simulink model "H250Model"  (R2022a)
settings: Solver=ode4  StartTime=0.0  StopTime=inf  FixedStep=Ts  RelTol=1e-3
values from neighbouring files (symbols this model uses):
  ModelFail_env_P_wind = [0 0 0]    [F450DegradedParamInit.m]    (also in H250DegradedParamInit.m; H250ModelParam4S.m; H333DegradedParamInit4S.m)
  ModelFail_motor_isEnable = 0    [F450DegradedParamInit.m]    (also in H250DegradedParamInit.m; H250ModelParam4S.m; H333DegradedParamInit4S.m)
  ModelFail_motor_kCt = [1 1 1 1 1 1 1 1]    [F450DegradedParamInit.m]    (also in H250DegradedParamInit.m; H250ModelParam4S.m; H333DegradedParamInit4S.m)
  ModelFail_motor_kTc = [1 1 1 1 1 1 1 1]    [F450DegradedParamInit.m]    (also in H250DegradedParamInit.m; H250ModelParam4S.m; H333DegradedParamInit4S.m)
  ModelFail_motor_kw = [1 1 1 1 1 1 1 1]    [F450DegradedParamInit.m]    (also in H250DegradedParamInit.m; H250ModelParam4S.m; H333DegradedParamInit4S.m)
  ModelInit_motorInitRate = 0    [F450DegradedParamInit.m]    (also in H250DegradedParamInit.m; H250ModelParam4S.m; H333DegradedParamInit4S.m)
  ModelParam_Airframe_CMP = [0 0 0]    [F450DegradedParamInit.m]    (also in H250DegradedParamInit.m; H250ModelParam4S.m; H333DegradedParamInit4S.m)
  ModelParam_Airframe_J = [0.0194 0 0;0 0.0194 0;0 0 0.0291]    [F450DegradedParamInit.m]    (also in H250DegradedParamInit.m = [0.0056 0 0;0 0.0056 0;0 0 0.0104]; H250ModelParam4S.m = [0.0056 0 0;0 0.0056 0;0 0 0.0104]; H333DegradedParamInit4S.m = [0.012 0 0;0 0.012 0;0 0 0.02])
  ModelParam_Airframe_m = 1.31    [F450DegradedParamInit.m]    (also in H250DegradedParamInit.m = 0.752; H250ModelParam4S.m = 0.71; H333DegradedParamInit4S.m = 1.13)
  ModelParam_envAltitude = 0    [F450DegradedParamInit.m]    (also in H250DegradedParamInit.m; H250ModelParam4S.m; H333DegradedParamInit4S.m)
  ModelParam_envC_d = 0.055    [F450DegradedParamInit.m]    (also in H250DegradedParamInit.m; H250ModelParam4S.m; H333DegradedParamInit4S.m)
  ModelParam_envC_md = [0.001 0.001 0.00058]    [F450DegradedParamInit.m]    (also in H250DegradedParamInit.m = [0.001 0.001 0.00040]; H250ModelParam4S.m = [0.001 0.001 0.0002]; H333DegradedParamInit4S.m = [0.001 0.001 0.0002])
  ModelParam_GPSEphFinal = 0.3    [F450DegradedParamInit.m]    (also in H250DegradedParamInit.m; H250ModelParam4S.m; H333DegradedParamInit4S.m)
  ModelParam_GPSEpvFinal = 0.4    [F450DegradedParamInit.m]    (also in H250DegradedParamInit.m; H250ModelParam4S.m; H333DegradedParamInit4S.m)
  ModelParam_GPSFix3DFix = 3    [F450DegradedParamInit.m]    (also in H250DegradedParamInit.m; H250ModelParam4S.m; H333DegradedParamInit4S.m)
  ModelParam_GPSSatsVisible = 10    [F450DegradedParamInit.m]    (also in H250DegradedParamInit.m; H250ModelParam4S.m; H333DegradedParamInit4S.m)
  ModelParam_motorCr = 842.1    [F450DegradedParamInit.m]    (also in H250DegradedParamInit.m = 0; H250ModelParam4S.m = 0; H333DegradedParamInit4S.m = 0)
  ModelParam_motorFitType = 1    [F450DegradedParamInit.m]    (also in H250DegradedParamInit.m = 2; H250ModelParam4S.m = 2; H333DegradedParamInit4S.m = 2)
  ModelParam_motorJm = 0.0000687    (= 6.87e-05)    [F450DegradedParamInit.m]    (also in H250DegradedParamInit.m = 8.8493e-06; H250ModelParam4S.m = 8.8493; H333DegradedParamInit4S.m = 8.8493e-06)
  ModelParam_motorMinThr = 0.05    [F450DegradedParamInit.m]    (also in H250DegradedParamInit.m = 0.148; H250ModelParam4S.m = 0.148; H333DegradedParamInit4S.m = 0.11)
  ModelParam_motorRateCurveCoeffi = [0 0 0]    [F450DegradedParamInit.m]    (also in H250DegradedParamInit.m = [-1364 3870 -372.4]; H250ModelParam4S.m = [-2143 5113 -458.4]; H333DegradedParamInit4S.m = [-1057 2662 -94.98])
  ModelParam_motorTc = 0.0214    [F450DegradedParamInit.m]    (also in H250DegradedParamInit.m = 0.035; H250ModelParam4S.m = 0.025; H333DegradedParamInit4S.m = 0.035)
  ModelParam_motorWb = 0    [F450DegradedParamInit.m]    (also in H250DegradedParamInit.m; H250ModelParam4S.m; H333DegradedParamInit4S.m)
  ModelParam_NoiseVarAcc0 = [0.1 0.1 0.1]    [F450DegradedParamInit.m]    (also in H250DegradedParamInit.m; H250ModelParam4S.m = [0.001 0.001 0.001]; H333DegradedParamInit4S.m)
  ModelParam_NoiseVarAcc1 = [0.1 0.1 0.1]    [F450DegradedParamInit.m]    (also in H250DegradedParamInit.m; H250ModelParam4S.m = [0.01 0.01 0.01]; H333DegradedParamInit4S.m)
  ModelParam_NoiseVarGPS_P0 = [1e-5 1e-5 1e-5]    [F450DegradedParamInit.m]    (also in H250DegradedParamInit.m; H250ModelParam4S.m; H333DegradedParamInit4S.m)
  ModelParam_NoiseVarGPS_V0 = [1e-5 1e-5 1e-5]    [F450DegradedParamInit.m]    (also in H250DegradedParamInit.m; H250ModelParam4S.m; H333DegradedParamInit4S.m)
  ModelParam_NoiseVarGyro0 = [0.0005 0.0005 0.0005]    [F450DegradedParamInit.m]    (also in H250DegradedParamInit.m; H250ModelParam4S.m = [0.00005 0.00005 0.00005]; H333DegradedParamInit4S.m)
  ModelParam_NoiseVarGyro1 = [0.004 0.004 0.004]    [F450DegradedParamInit.m]    (also in H250DegradedParamInit.m; H250ModelParam4S.m; H333DegradedParamInit4S.m)
  ModelParam_NoiseVarMag0 = [0.000002 0.000002 0.000002]    [F450DegradedParamInit.m]    (also in H250DegradedParamInit.m; H250ModelParam4S.m; H333DegradedParamInit4S.m)
  ModelParam_NoiseVarMag1 = [0.0001 0.0001 0.0001]    [F450DegradedParamInit.m]    (also in H250DegradedParamInit.m; H250ModelParam4S.m; H333DegradedParamInit4S.m)
  ModelParam_PositionAcc0 = [0.071  0  -0.1365]    [F450DegradedParamInit.m]    (also in H250DegradedParamInit.m; H250ModelParam4S.m; H333DegradedParamInit4S.m)
  ModelParam_PositionAcc1 = [0.071  0  -0.1365]    [F450DegradedParamInit.m]    (also in H250DegradedParamInit.m; H250ModelParam4S.m; H333DegradedParamInit4S.m)
  ModelParam_rotorCt = 1.681e-05    [F450DegradedParamInit.m]    (also in H250DegradedParamInit.m = 1.448e-06; H250ModelParam4S.m = 1.345; H333DegradedParamInit4S.m = 7.586e-06)
  ModelParam_WalkNoiseVarAcc0 = [0.001 0.001 0.001]    [F450DegradedParamInit.m]    (also in H250DegradedParamInit.m; H250ModelParam4S.m = [0.0001 0.0001 0.0001]; H333DegradedParamInit4S.m)
  ModelParam_WalkNoiseVarAcc1 = [0.001 0.001 0.001]    [F450DegradedParamInit.m]    (also in H250DegradedParamInit.m; H250ModelParam4S.m; H333DegradedParamInit4S.m)
  ModelParam_WalkNoiseVarGPS_P0 = [0.01 0.01 0.01]    [F450DegradedParamInit.m]    (also in H250DegradedParamInit.m; H250ModelParam4S.m = [0 0 0]; H333DegradedParamInit4S.m)
  ModelParam_WalkNoiseVarGPS_V0 = [0.01 0.01 0.01]    [F450DegradedParamInit.m]    (also in H250DegradedParamInit.m; H250ModelParam4S.m = [0 0 0]; H333DegradedParamInit4S.m)
  ModelParam_WalkNoiseVarGyro0 = [0.00004 0.00004 0.00004]    [F450DegradedParamInit.m]    (also in H250DegradedParamInit.m; H250ModelParam4S.m; H333DegradedParamInit4S.m)
  ModelParam_WalkNoiseVarGyro1 = [0.00004 0.00004 0.00004]    [F450DegradedParamInit.m]    (also in H250DegradedParamInit.m; H250ModelParam4S.m; H333DegradedParamInit4S.m)
  ModelParam_WalkNoiseVarMag0 = [0.000001 0.000001 0.000001]    [F450DegradedParamInit.m]    (also in H250DegradedParamInit.m; H250ModelParam4S.m; H333DegradedParamInit4S.m)
  ModelParam_WalkNoiseVarMag1 = [0.000001 0.000001 0.000001]    [F450DegradedParamInit.m]    (also in H250DegradedParamInit.m; H250ModelParam4S.m; H333DegradedParamInit4S.m)
  MulticopterLayoutConfig = 1    [F450DegradedParamInit.m]    (also in H250DegradedParamInit.m = 6; H250ModelParam4S.m = 7; H333DegradedParamInit4S.m = 8)
  RflySimDisplayUAVType = 3    [F450DegradedParamInit.m]    (also in H250DegradedParamInit.m; H250ModelParam4S.m; H333DegradedParamInit4S.m)
  Ts = 1/1000    (= 0.001)    [F450DegradedParamInit.m]    (also in H250DegradedParamInit.m; H250ModelParam4S.m; H333DegradedParamInit4S.m)
undefined symbols (not defined in the file or in its folder): Earth, WGS84
libraries: aerolibnav x5, aerolibtransform2 x3, sharedtransform x3, aerolibutil x2, sharedutil x1, shared6dof x1, aerolibasang x1, aerolibatmos2 x1, aerolibconvert2 x1
(part 3 of 3)

== system H250Model/ESC&Motor Model/MotorNonlinearDynamic4/MotorDynamic ==
  ReferenceRate : Inport  Unit=rad/s
  MotorInitRate : Inport  Port=2  Unit=rad/s
  MotorTimeConstant : Inport  Port=3  Unit=s
  Divide : Product  Inputs=*/
  Integrator : Integrator  InitialConditionSource=external
  Sum : Sum  Inputs=-+|
  MotorRate : Outport  Unit=rad/s
  wires:
  MotorInitRate/1 -> Integrator/2
  Integrator/1 -> Sum/1, MotorRate/1
  Divide/1 -> Integrator/1
  MotorTimeConstant/1 -> Divide/2
  Sum/1 -> Divide/1
  ReferenceRate/1 -> Sum/2

== system H250Model/ESC&Motor Model/MotorNonlinearDynamic5/MotorDynamic ==
  ReferenceRate : Inport  Unit=rad/s
  MotorInitRate : Inport  Port=2  Unit=rad/s
  MotorTimeConstant : Inport  Port=3  Unit=s
  Divide : Product  Inputs=*/
  Integrator : Integrator  InitialConditionSource=external
  Sum : Sum  Inputs=-+|
  MotorRate : Outport  Unit=rad/s
  wires:
  ReferenceRate/1 -> Sum/2
  Sum/1 -> Divide/1
  MotorTimeConstant/1 -> Divide/2
  Divide/1 -> Integrator/1
  Integrator/1 -> MotorRate/1, Sum/1
  MotorInitRate/1 -> Integrator/2

== system H250Model/ESC&Motor Model/MotorNonlinearDynamic6/MotorDynamic ==
  ReferenceRate : Inport  Unit=rad/s
  MotorInitRate : Inport  Port=2  Unit=rad/s
  MotorTimeConstant : Inport  Port=3  Unit=s
  Divide : Product  Inputs=*/
  Integrator : Integrator  InitialConditionSource=external
  Sum : Sum  Inputs=-+|
  MotorRate : Outport  Unit=rad/s
  wires:
  MotorInitRate/1 -> Integrator/2
  Integrator/1 -> Sum/1, MotorRate/1
  Divide/1 -> Integrator/1
  MotorTimeConstant/1 -> Divide/2
  Sum/1 -> Divide/1
  ReferenceRate/1 -> Sum/2

== system H250Model/ESC&Motor Model/MotorNonlinearDynamic7/MotorDynamic ==
  ReferenceRate : Inport  Unit=rad/s
  MotorInitRate : Inport  Port=2  Unit=rad/s
  MotorTimeConstant : Inport  Port=3  Unit=s
  Divide : Product  Inputs=*/
  Integrator : Integrator  InitialConditionSource=external
  Sum : Sum  Inputs=-+|
  MotorRate : Outport  Unit=rad/s
  wires:
  ReferenceRate/1 -> Sum/2
  Sum/1 -> Divide/1
  MotorTimeConstant/1 -> Divide/2
  Divide/1 -> Integrator/1
  Integrator/1 -> MotorRate/1, Sum/1
  MotorInitRate/1 -> Integrator/2

== system H250Model/ESC&Motor Model/MotorNonlinearDynamic8/MotorDynamic ==
  ReferenceRate : Inport  Unit=rad/s
  MotorInitRate : Inport  Port=2  Unit=rad/s
  MotorTimeConstant : Inport  Port=3  Unit=s
  Divide : Product  Inputs=*/
  Integrator : Integrator  InitialConditionSource=external
  Sum : Sum  Inputs=-+|
  MotorRate : Outport  Unit=rad/s
  wires:
  MotorInitRate/1 -> Integrator/2
  Integrator/1 -> Sum/1, MotorRate/1
  Divide/1 -> Integrator/1
  MotorTimeConstant/1 -> Divide/2
  Sum/1 -> Divide/1
  ReferenceRate/1 -> Sum/2

== matlab function H250Model/ESC&Motor Model/MotorNonlinearDynamic5/ESC_MotorSteadyState ==
  data: Throttle input; BatteryEfficiency input; SteadyStateRate output; Cr input; Ratebias input; MotorMinThr parameter; MotorRateCurveCoeffi input; MotorFitType input
function SteadyStateRate = ESC_MotorSteadyState(Throttle, BatteryEfficiency, Cr, Ratebias, MotorMinThr, MotorRateCurveCoeffi, MotorFitType)
if MotorFitType ==1
    %线性拟合则采用如下计算
    if Throttle>1
        Throttle = 1;
    end
    if Throttle<MotorMinThr
        SteadyStateRate = 0.0;
    else
        SteadyStateRate = Cr*BatteryEfficiency*Throttle + Ratebias;
    end
    
else
    %二次拟合则采用如下计算
    if Throttle>1
        Throttle = 1;
    end
    if Throttle<MotorMinThr
        SteadyStateRate = 0.0;
    else    
        SteadyStateRate = MotorRateCurveCoeffi(1)*(BatteryEfficiency*Throttle)^2 + MotorRateCurveCoeffi(2)*BatteryEfficiency*Throttle + MotorRateCurveCoeffi(3);
    end
    
end

== matlab function H250Model/Environment Model/Ground Model/OnGroundFaceup ==
  data: EulerAng input; y output
function y = fcn(EulerAng)

targetRoll = 0;
% if cos(EulerAng(1))<0
%     targetRoll=pi;  
% end

targetPitch = 0;
% if cos(EulerAng(2))<0
%         targetPitch=pi;
% end
    
y = [targetRoll;targetPitch;EulerAng(3)];

== matlab function H250Model/ESC&Motor Model/Concatenate Motor Input ==
  data: inPWMs input; motorIn output; BatteryEfficiency input; kw input; kTc input; kCt input; isEnable input
function motorIn  = fcn(inPWMs, BatteryEfficiency, kw, kTc, kCt, isEnable)
if isEnable
motorIn = [inPWMs'; 
 [BatteryEfficiency, BatteryEfficiency, BatteryEfficiency, BatteryEfficiency, BatteryEfficiency, BatteryEfficiency, BatteryEfficiency, BatteryEfficiency];
 kw' ;
 kTc' ;
 kCt'];
else
motorIn = [inPWMs'; 
 [1  1  1  1  1  1  1  1];
 [1  1  1  1  1  1  1  1] ;
 [1  1  1  1  1  1  1  1] ;
 [1  1  1  1  1  1  1  1] ];
end

== matlab function H250Model/ESC&Motor Model/MotorNonlinearDynamic6/ESC_MotorSteadyState ==
  data: Throttle input; BatteryEfficiency input; SteadyStateRate output; Cr input; Ratebias input; MotorMinThr parameter; MotorRateCurveCoeffi input; MotorFitType input
function SteadyStateRate = ESC_MotorSteadyState(Throttle, BatteryEfficiency, Cr, Ratebias, MotorMinThr, MotorRateCurveCoeffi, MotorFitType)
if MotorFitType ==1
    %线性拟合则采用如下计算
    if Throttle>1
        Throttle = 1;
    end
    if Throttle<MotorMinThr
        SteadyStateRate = 0.0;
    else
        SteadyStateRate = Cr*BatteryEfficiency*Throttle + Ratebias;
    end
    
else
    %二次拟合则采用如下计算
    if Throttle>1
        Throttle = 1;
    end
    if Throttle<MotorMinThr
        SteadyStateRate = 0.0;
    else    
        SteadyStateRate = MotorRateCurveCoeffi(1)*(BatteryEfficiency*Throttle)^2 + MotorRateCurveCoeffi(2)*BatteryEfficiency*Throttle + MotorRateCurveCoeffi(3);
    end
    
end

== matlab function H250Model/ESC&Motor Model/MotorNonlinearDynamic7/ESC_MotorSteadyState ==
  data: Throttle input; BatteryEfficiency input; SteadyStateRate output; Cr input; Ratebias input; MotorMinThr parameter; MotorRateCurveCoeffi input; MotorFitType input
function SteadyStateRate = ESC_MotorSteadyState(Throttle, BatteryEfficiency, Cr, Ratebias, MotorMinThr, MotorRateCurveCoeffi, MotorFitType)
if MotorFitType ==1
    %线性拟合则采用如下计算
    if Throttle>1
        Throttle = 1;
    end
    if Throttle<MotorMinThr
        SteadyStateRate = 0.0;
    else
        SteadyStateRate = Cr*BatteryEfficiency*Throttle + Ratebias;
    end
    
else
    %二次拟合则采用如下计算
    if Throttle>1
        Throttle = 1;
    end
    if Throttle<MotorMinThr
        SteadyStateRate = 0.0;
    else    
        SteadyStateRate = MotorRateCurveCoeffi(1)*(BatteryEfficiency*Throttle)^2 + MotorRateCurveCoeffi(2)*BatteryEfficiency*Throttle + MotorRateCurveCoeffi(3);
    end
    
end

== matlab function H250Model/ESC&Motor Model/MotorNonlinearDynamic8/ESC_MotorSteadyState ==
  data: Throttle input; BatteryEfficiency input; SteadyStateRate output; Cr input; Ratebias input; MotorMinThr parameter; MotorRateCurveCoeffi input; MotorFitType input
function SteadyStateRate = ESC_MotorSteadyState(Throttle, BatteryEfficiency, Cr, Ratebias, MotorMinThr, MotorRateCurveCoeffi, MotorFitType)
if MotorFitType ==1
    %线性拟合则采用如下计算
    if Throttle>1
        Throttle = 1;
    end
    if Throttle<MotorMinThr
        SteadyStateRate = 0.0;
    else
        SteadyStateRate = Cr*BatteryEfficiency*Throttle + Ratebias;
    end
    
else
    %二次拟合则采用如下计算
    if Throttle>1
        Throttle = 1;
    end
    if Throttle<MotorMinThr
        SteadyStateRate = 0.0;
    else    
        SteadyStateRate = MotorRateCurveCoeffi(1)*(BatteryEfficiency*Throttle)^2 + MotorRateCurveCoeffi(2)*BatteryEfficiency*Throttle + MotorRateCurveCoeffi(3);
    end
    
end

== matlab function H250Model/Environment Model/MATLAB Function ==
  data: g input; m input; F_env output; Vb input; Wb input; DCM input; M_env output; C_d input; C_md input; P_wind input
function [F_env, M_env] = fcn(g, m, Vb, Wb, DCM, C_d, C_md, P_wind)
% 计算空气流动产生的力,这里的F_env其实就是空气阻力F_d 或者说F_wind
F_wind = -C_d * Vb.*abs(Vb);
% 考虑重力场产生的重力
F_env = F_wind + DCM*m*g;

% 计算转动阻尼力矩
M_d = -C_md.* Wb.*abs(Wb);
% 计算空气阻力产生的力矩
M_wind = cross(P_wind, F_wind);
M_env = M_wind + M_d;

== matlab function H250Model/Sensor Model/Barometer/Pressure Function ==
  data: h input; p output
function p = fcn(h)
% R 普适用气体常量8.31
% miu 空气摩尔质量 28.959
% T0 零海拔气温（K）
% n 或者 r 表示多方指数 范围1-1.4  一般取1.235
% g 重力加速度 9.8
p=((1-h/0.3048/145366.45))^(1/0.190284)*101325;

== matlab function H250Model/Sensor Model/Magnetometer Hub/MATLAB Function ==
  data: DCM input; mag_e input; b_m input; n_m input; Mag_means output; K_m input
function Mag_means = fcn(DCM, mag_e, b_m, n_m, K_m)
 
Mag_means = K_m*DCM*mag_e + b_m + n_m;

== matlab function H250Model/Sensor Model/Magnetometer Hub/MATLAB Function1 ==
  data: DCM input; mag_e input size=3; b_m input size=3; n_m input size=3; Mag_means output size=3; K_m input
function Mag_means = fcn(DCM, mag_e, b_m, n_m, K_m)
 
Mag_means = K_m*DCM*mag_e + b_m + n_m;

== matlab function H250Model/Sensor Model/GPS/GenCogVel ==
  data: vel output; Ve input; cot output
function [vel,cot] = Ang360(Ve)
vel=norm(Ve(1:2));

if vel < 1
    cot = 0;
else
    cot=atan2d(Ve(2),Ve(1));
end
 
if cot<0
    cot=cot+360;
end

== matlab function H250Model/Force and Moment Model/Allocation Model/Efficiency Function ==
  data: index input; EfficiencyMatrix output; o_m input; RotorDirectionVector output
function [EfficiencyMatrix, RotorDirectionVector] = EfficiencyFcn(index,o_m)
% index 动力布局配置序号
% o_m   质心位于非质心机体系中的坐标
% EfficiencyMatrix 选中的动力布局下的控制效率矩阵
%% 动力布局配置（本节用户可根据需要增加配置）
% 动力系统布局配置有两种配置方法，采用结构体的方式表示
% 结构体中包好两个成员分别是 Type Matrix
% #第一种：结构体中成员Type值为1
    % 数组中列号表示飞控所对应的电机序号。
    % 例如飞控输出的1号电机控制量对应数组中第一列的参数

    % 第一行表示：电机旋转方向，俯视时，顺时针为 -1 逆时针为 +1 
    % 第二行表示：机臂在机体坐标系下的方位角 
    % 第三行表示：机臂长度
    % 第四行表示：反扭力矩系数与拉力系数之比
% #第二种：结构体中成员Type值为2
    % 第二种方法需要提供机臂在 非质心机体系中的坐标，以及质心在非质心机体系中的坐标。
    % 非质心机体系的原点可以与质心重合，也可以不重合，
    % 此举是为了便于表述质心变化对力臂产生的影响，
    % 力臂的长度会随着质心的变化而变化，但是机臂对于机体却是固定的。
    % 所以需要选取一非质心（例如形心）坐标系与机体固连确保对于机臂和质心的位置描述是固定的。机体非质心坐标系正方向应该与NED对应。
    
    % 配置矩阵为5x8大小，8列代表八个旋翼，本模型目前按照最多8个旋翼来设计
    % 列号对应飞控输出的电机序号，例如第一列就是飞控中PWM1的输出对应的电机。
    % 也就是说即使都是六轴，那么如果不同的飞控对于电机序号对应的位置定义各不同的话，那么就应该对应不同的动力布局配置。
    % 第一行表示：电机旋转方向，俯视时，顺时针为 -1 逆时针为 +1
    % 第二行到第四行分别表示：机臂坐标的x、y、z单位为m
    % 第五行表示：反扭力矩系数与拉力系数之比 $c_M/c_T$
% 动力布局配置 1:X F450
Config1.Type = 1;
Config1.Matrix = [1 1 -1 -1 0 0 0 0;
                 pi/4 pi/4+pi pi/4+3*pi/2 pi/4+pi/2 0 0 0 0;
                 0.225 0.225 0.225 0.225 0 0 0 0;
                 0.0166 0.0166 0.0166 0.0166 0 0 0 0];
% 动力布局配置 2:+ F450
Config2.Type = 1;
Config2.Matrix = [1 -1 1 -1 0 0 0 0;
                 pi/2 pi 3*pi/2 0  0 0 0 0;
                 0.255 0.255 0.255 0.255 0 0 0 0;
                 0.0166 0.0166 0.0166 0.0166 0 0 0 0];
% 动力布局配置 3:+ F450 配合PX4 +控制器
Config3.Type = 1;
Config3.Matrix = [1 1 -1 -1 0 0 0 0;
                   pi/2 1.5*pi 0 pi 0 0 0 0;
                   0.225 0.225 0.225 0.225 0 0 0 0;
                   0.0166 0.0166 0.0166 0.0166 0 0 0 0];
% 动力布局配置 4 美团六轴
Config4.Type = 2;
Config4.Matrix =[-1             1              -1               1                1               -1                 0 0;
                             0              0               0.405       -0.390         0.405        -0.390           0 0;
                             0.366     -0.366       -0.28722     0.28722     0.28722    -0.28722      0 0;
                             0.046       0.046       -0.046       -0.046        -0.046       -0.046           0 0;
                            1.924e-2  1.924e-2   1.924e-2   1.924e-2     1.924e-2   1.924e-2       0 0];
% 动力布局配置 5 HIL测试六轴
Config5.Type = 1;
Config5.Matrix = [-1                1                  -1                1                   1             -1                 0  0;
                              90*pi/180   270*pi/180   330*pi/180  150*pi/180  30*pi/180      210*pi/180  0 0;
                               0.366         0.366           0.366          0.366            0.366       0.366           0 0;
                               0.016         0.016            0.016         0.016            0.016       0.016           0 0];
                           
% 动力布局配置 6:X H250 12V 电机序号顺序：对角线
Config6.Type = 1;
Config6.Matrix = [1 1 -1 -1 0 0 0 0;
                 pi/4 pi/4+pi pi/4+3*pi/2 pi/4+pi/2 0 0 0 0;
                 0.125 0.125 0.125 0.125 0 0 0 0;
                 0.0154 0.0154 0.0154 0.0154 0 0 0 0];

% 动力布局配置 7:X H250 4S 电机序号顺序：对角线
Config7.Type = 1;
Config7.Matrix = [1 1 -1 -1 0 0 0 0;
                 pi/4 pi/4+pi pi/4+3*pi/2 pi/4+pi/2 0 0 0 0;
                 0.125 0.125 0.125 0.125 0 0 0 0;
                 0.0166 0.0166 0.0166 0.0166 0 0 0 0];
             
 % 动力布局配置 8:X H333 4S 电机序号顺序：对角线
Config8.Type = 1;
Config8.Matrix = [1 1 -1 -1 0 0 0 0;
                 pi/4 pi/4+pi pi/4+3*pi/2 pi/4+pi/2 0 0 0 0;
                 0.1665 0.1665 0.1665 0.1665 0 0 0 0;
                 0.0165 0.0165 0.0165 0.0165 0 0 0 0];
             
% 构建结构体数组，便于检索，举例如果要增加配置需要做如下修改
% 假如原代码为   Config = [Config1 Config2 Config3 Config4]; 
% 新增了Config5 
% 那么代码修改为Config = [Config1 Config2 Config3 Config4 Config5];
Config = [Config1 Config2 Config3 Config4 Config5 Config6 Config7 Config8];
%% 选取配置
ConfigCurrent = Config(index);
if ConfigCurrent.Type ==1
    Matrix = [  0 0 0 0 0 0 0 0;
                      0 0 0 0 0 0 0 0;
                    -1 -1 -1 -1 -1 -1 -1  -1;
                    -ConfigCurrent.Matrix(3,:).* sin(ConfigCurrent.Matrix(2,:));
                    ConfigCurrent.Matrix(3,:).* cos(ConfigCurrent.Matrix(2,:));
                    ConfigCurrent.Matrix(4,:).* ConfigCurrent.Matrix(1,:)];
    Vector = ConfigCurrent.Matrix(1,:);
else
    Matrix = [  0 0 0 0 0 0 0 0;
                      0 0 0 0 0 0 0 0;
                    -1 -1 -1 -1 -1 -1 -1  -1;
                    -(ConfigCurrent.Matrix(3,:)-o_m(2));
                    ConfigCurrent.Matrix(2,:)-o_m(1);
                    ConfigCurrent.Matrix(5,:).* ConfigCurrent.Matrix(1,:)];
    Vector = ConfigCurrent.Matrix(1,:);
end
EfficiencyMatrix = Matrix;
RotorDirectionVector = Vector;

== matlab function H250Model/Environment Model/Ground Model/Ground Model ==
  settings: updateMethod=DISCRETE
  data: mg input; wb input; Xe input; F1 output; Ve input; M1 output; Quet input; terrainZ input; landed output; takeoff output
function [F1,M1,landed,takeoff] = fcn(mg,wb,Xe,Ve,Quet,terrainZ)
% This is a ground model that can provides reaction force and reaction torque

% persistent z0;
% if isempty(z0)
%      z0=0;
% end

persistent takeoffFlag;
if isempty(takeoffFlag)
     takeoffFlag=int8(0);
end

persistent landFlag;
if isempty(landFlag)
     landFlag=int8(1);
end


z=Xe(3)-terrainZ;

 if (z<-0.3)&&(Ve(3)<-0.1)&&(takeoffFlag<0.5)
    takeoffFlag=int8(1);
    landFlag=int8(0);
 end
 
 if (z>-0.05)&&(Ve(3)>0.1)&&(landFlag<0.5)
    landFlag=int8(1);
    takeoffFlag=int8(0);
    %z0=terrainZ;
 end

takeoff = takeoffFlag;
landed = landFlag;


F1=[0;0;0];
M1=[0;0;0];

if z>=0
%     if z>=0.3
%         if Ve(3)>=5
%             F1(3)=-mg(3)-1000*Ve(3);
%         else
%             F1(3)=-mg(3)-500*z-100*Ve(3);  
%         end
%     elseif z>=0.1
%         if Ve(3)>=2
%             F1(3)=-mg(3)-100*Ve(3);
%         else
%             F1(3)=-mg(3)-50*z-100*Ve(3);  
%         end
%     else
%          if Ve(3)>=1
%             F1(3)=-mg(3)-50*Ve(3);
%         else
%             F1(3)=-mg(3)-5*z-50*Ve(3);  
%         end       
%     end
    if z<0.05
         F1(3)=-mg(3)-10*Ve(3); 
    elseif z<0.1
        F1(3)=-mg(3)-0.5*z-20*Ve(3); 
    else
         F1(3)=-mg(3)-1*z-50*Ve(3); 
    end

    
    F1(1)=-50*Ve(1);
    F1(2)=-50*Ve(2);
    M1=-20*[Quet(2);Quet(3);Quet(4)]-5*wb;
    M1 = M1 * abs(mg(3))*0.0333;
end

== matlab function H250Model/ESC&Motor Model/MotorNonlinearDynamic2/ESC_MotorSteadyState ==
  data: Throttle input; BatteryEfficiency input; SteadyStateRate output; Cr input; Ratebias input; MotorMinThr parameter; MotorRateCurveCoeffi input; MotorFitType input
function SteadyStateRate = ESC_MotorSteadyState(Throttle, BatteryEfficiency, Cr, Ratebias, MotorMinThr, MotorRateCurveCoeffi, MotorFitType)
if MotorFitType ==1
    %线性拟合则采用如下计算
    if Throttle>1
        Throttle = 1;
    end
    if Throttle<MotorMinThr
        SteadyStateRate = 0.0;
    else
        SteadyStateRate = Cr*BatteryEfficiency*Throttle + Ratebias;
    end
    
else
    %二次拟合则采用如下计算
    if Throttle>1
        Throttle = 1;
    end
    if Throttle<MotorMinThr
        SteadyStateRate = 0.0;
    else    
        SteadyStateRate = MotorRateCurveCoeffi(1)*(BatteryEfficiency*Throttle)^2 + MotorRateCurveCoeffi(2)*BatteryEfficiency*Throttle + MotorRateCurveCoeffi(3);
    end
    
end

== matlab function H250Model/ESC&Motor Model/MotorNonlinearDynamic1/ESC_MotorSteadyState ==
  data: Throttle input; BatteryEfficiency input; SteadyStateRate output; Cr input; Ratebias input; MotorMinThr parameter; MotorRateCurveCoeffi input; MotorFitType input
function SteadyStateRate = ESC_MotorSteadyState(Throttle, BatteryEfficiency, Cr, Ratebias, MotorMinThr, MotorRateCurveCoeffi, MotorFitType)
if MotorFitType ==1
    %线性拟合则采用如下计算
    if Throttle>1
        Throttle = 1;
    end
    if Throttle<MotorMinThr
        SteadyStateRate = 0.0;
    else
        SteadyStateRate = Cr*BatteryEfficiency*Throttle + Ratebias;
    end
    
else
    %二次拟合则采用如下计算
    if Throttle>1
        Throttle = 1;
    end
    if Throttle<MotorMinThr
        SteadyStateRate = 0.0;
    else    
        SteadyStateRate = MotorRateCurveCoeffi(1)*(BatteryEfficiency*Throttle)^2 + MotorRateCurveCoeffi(2)*BatteryEfficiency*Throttle + MotorRateCurveCoeffi(3);
    end
    
end

== matlab function H250Model/ESC&Motor Model/MotorNonlinearDynamic3/ESC_MotorSteadyState ==
  data: Throttle input; BatteryEfficiency input; SteadyStateRate output; Cr input; Ratebias input; MotorMinThr parameter; MotorRateCurveCoeffi input; MotorFitType input
function SteadyStateRate = ESC_MotorSteadyState(Throttle, BatteryEfficiency, Cr, Ratebias, MotorMinThr, MotorRateCurveCoeffi, MotorFitType)
if MotorFitType ==1
    %线性拟合则采用如下计算
    if Throttle>1
        Throttle = 1;
    end
    if Throttle<MotorMinThr
        SteadyStateRate = 0.0;
    else
        SteadyStateRate = Cr*BatteryEfficiency*Throttle + Ratebias;
    end
    
else
    %二次拟合则采用如下计算
    if Throttle>1
        Throttle = 1;
    end
    if Throttle<MotorMinThr
        SteadyStateRate = 0.0;
    else    
        SteadyStateRate = MotorRateCurveCoeffi(1)*(BatteryEfficiency*Throttle)^2 + MotorRateCurveCoeffi(2)*BatteryEfficiency*Throttle + MotorRateCurveCoeffi(3);
    end
    
end

== matlab function H250Model/ESC&Motor Model/MotorNonlinearDynamic4/ESC_MotorSteadyState ==
  data: Throttle input; BatteryEfficiency input; SteadyStateRate output; Cr input; Ratebias input; MotorMinThr parameter; MotorRateCurveCoeffi input; MotorFitType input
function SteadyStateRate = ESC_MotorSteadyState(Throttle, BatteryEfficiency, Cr, Ratebias, MotorMinThr, MotorRateCurveCoeffi, MotorFitType)
if MotorFitType ==1
    %线性拟合则采用如下计算
    if Throttle>1
        Throttle = 1;
    end
    if Throttle<MotorMinThr
        SteadyStateRate = 0.0;
    else
        SteadyStateRate = Cr*BatteryEfficiency*Throttle + Ratebias;
    end
    
else
    %二次拟合则采用如下计算
    if Throttle>1
        Throttle = 1;
    end
    if Throttle<MotorMinThr
        SteadyStateRate = 0.0;
    else    
        SteadyStateRate = MotorRateCurveCoeffi(1)*(BatteryEfficiency*Throttle)^2 + MotorRateCurveCoeffi(2)*BatteryEfficiency*Throttle + MotorRateCurveCoeffi(3);
    end
    
end
